simulink model "unloaded_motor"  (R2021b)
settings: Solver=VariableStepAuto  StartTime=0.0  StopTime=0.01  RelTol=1e-3
undefined symbols (not defined in the file or in its folder): Km, TCspd, Ym
libraries: cstblocks x2
settings Model: Creator=andre  LastModifiedBy=andre

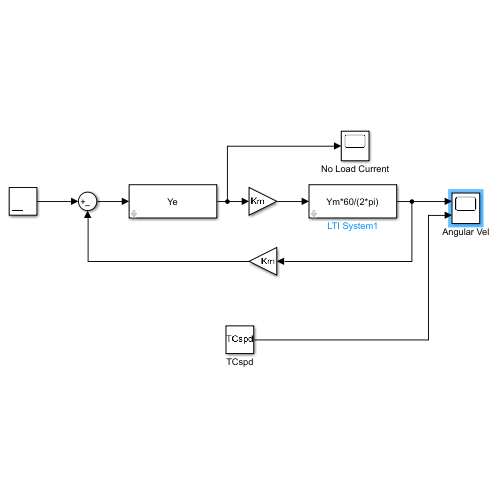
[thumbnail: Simulink's stored preview of the top-level diagram]
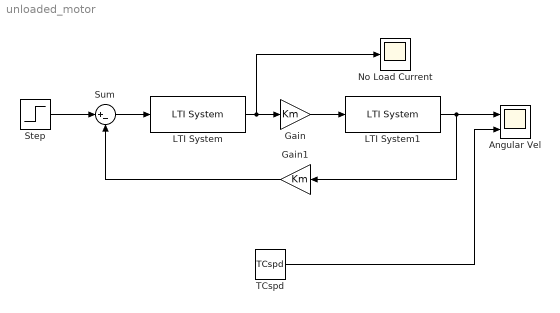
== system unloaded_motor ==
  Angular Vel : Scope  NumInputPorts=2
  Gain : Gain  Gain=Km
  Gain1 : Gain  Gain=Km
  LTI System : cstblocks/LTI System  sys=Ye  IC=[]
  LTI System1 : cstblocks/LTI System  sys=Ym*60/(2*pi)  IC=[]
  No Load Current : Scope
  Step : Step  Time=0  After=12  SampleTime=0
  Sum : Sum  Inputs=|+-
  TCspd : Constant  Value=TCspd
  wires:
  LTI System/1 -> No Load Current/1, Gain/1
  Gain/1 -> LTI System1/1
  LTI System1/1 -> Gain1/1, Angular Vel/1
  Step/1 -> Sum/1
  Gain1/1 -> Sum/2
  Sum/1 -> LTI System/1
  TCspd/1 -> Angular Vel/2
